simulink model "torqueBalancingStandup"  (Simulink 8.8)
settings: Solver=FixedStepDiscrete  StartTime=0.0  StopTime="Config.SIMULATION_TIME "  FixedStep=Config.Ts  RelTol=1e-3  EnableMultiTasking=on
InitFcn:
  | cd(fileparts(which(bdroot)));
  | initTorqueBalancingStandup;
StopFcn:
  | cd(fileparts(which(bdroot)));
  | stopTorqueBalancingStandup;
undefined symbols (not defined in the file or in its folder): bVectorConstraintsFeet, bVectorConstraintsLegs, Config, ConstraintsMatrixFeet, ConstraintsMatrixLegs, Gain, HUMAN_DOF_FOR_SIMULINK, Reg, ROBOT_DOF, ROBOT_DOF_FOR_SIMULINK, Sat, Sm
libraries: WBToolboxLibrary x128, simulink x4
(part 3 of 3)

== matlab function Robot System/Robot State and References/State Machine Standup/Compute base to fixed link transform/LFoot to base link transform /fromImuToHomogeousTransformFCN ==
  data: imu_H_link input double; imu_H_link_0 input double; link_H_base input double; inertial_0 input double; inertial input double; neck_pos input double; w_H_b output double; Config parameter double
function w_H_b = worldToBaseTransformWithIMUFCN(imu_H_link,imu_H_link_0,link_H_base,inertial_0,inertial,neck_pos,Config)

    w_H_b = worldToBaseTransformWithIMU(imu_H_link,imu_H_link_0,link_H_base,inertial_0,inertial,neck_pos,Config);

end

== matlab function Robot System/Dynamics and Kinematics/Kinematics/Legs in Contact ==
  data: icubStandup input double; legsInContact output double; state input double
function legsInContact = legsContactDetectorFCN(icubStandup,state)

   legsInContact = legsContactDetector(icubStandup,state);
end

== matlab function Robot System/Robot State and References/Internal Coordinator/Reference Generator CoM ==
  data: pos_CoM_0 input double; t input double; references_CoM output double; Config parameter double
function references_CoM = referenceGeneratorCoMFCN(pos_CoM_0, t, Config)

    references_CoM = referenceGeneratorCoM(pos_CoM_0, t, Config);
end

== matlab function Robot System/controller_QP/Compute angular momentum integral/Legs in Contact ==
  data: icubStandup input double; legsInContact output double; state input double
function legsInContact = legsContactDetectorFCN(icubStandup,state)

   legsInContact = legsContactDetector(icubStandup,state);
end

== matlab function Robot System/robot world to human feet transformation/MATLAB Function ==
  data: w_H_humanLeftFeet output double; w_H_robotLeftFeet input double; w_H_robotRightFeet input double; w_H_humanRightFeet output double
function [w_H_humanLeftFeet, w_H_humanRightFeet ]= fcn(w_H_robotLeftFeet,w_H_robotRightFeet)

    %% Fixed transformation from the robot feet to human feet defined
    %  human-forces-provider module configuration
    robotLeftFeet_H_humanLeftFeet = [-1.0   0.0     0.0     0.59;
                                      0.0  -1.0     0.0    -0.2549;
                                      0.0   0.0     1.0     0.0;
                                      0.0   0.0     0.0     1.0];
                                  
    robotRightFeet_H_humanRightFeet = [-1.0   0.0     0.0     0.59;
                                        0.0  -1.0     0.0    -0.2549;
                                        0.0   0.0     1.0     0.0;
                                        0.0   0.0     0.0     1.0];
                                  
    w_H_humanLeftFeet  = w_H_robotLeftFeet * robotLeftFeet_H_humanLeftFeet;
    
    w_H_humanRightFeet = w_H_robotRightFeet * robotRightFeet_H_humanRightFeet;

end

== matlab function Robot System/Robot State and References/State Machine Standup/stateMachineStandupFCN ==
  data: wrench_rightFoot input double; wrench_leftFoot input double; w_H_b output double; constraints output double; CoM_des output double; qj_des output double; wrench_leftHand input double; wrench_rightHand input double; xCoM_0 input double; qj_0 input double; xCoM input double; l_sole_H_b input double; l_upper_leg_contact_H_b input double; t input double; STANDUP_WITH_HUMAN_FORCE input double; STANDUP_WITH_HUMAN_TORQUE input double; Sm parameter double; impedances output double; KPCoM output double; KDCoM output double; Gain parameter double; currentState output double; jointsAndCoMSmoothingTime output double; fArms_phri input double
function [w_H_b, constraints, CoM_des, qj_des, impedances, KPCoM, KDCoM, currentState, jointsAndCoMSmoothingTime] = ...
             stateMachineStandupFCN(wrench_rightFoot, wrench_leftFoot, wrench_leftHand, wrench_rightHand, xCoM_0, qj_0, xCoM, l_sole_H_b, l_upper_leg_contact_H_b, t, STANDUP_WITH_HUMAN_FORCE, STANDUP_WITH_HUMAN_TORQUE, Sm, Gain, fArms_phri)
         
         [w_H_b, constraints, CoM_des, qj_des, impedances, KPCoM, KDCoM, currentState, jointsAndCoMSmoothingTime] = ...
             stateMachineStandup(wrench_rightFoot, wrench_leftFoot, wrench_leftHand, wrench_rightHand, xCoM_0, qj_0, xCoM, l_sole_H_b, l_upper_leg_contact_H_b, t, STANDUP_WITH_HUMAN_FORCE, STANDUP_WITH_HUMAN_TORQUE, Sm, Gain, fArms_phri);
end

== matlab function Robot System/Robot State and References/State Machine Standup/Compute State Velocity/Fixed Links Jacobians/Legs in Contact ==
  data: icubStandup input double; legsInContact output double; state input double
function legsInContact = legsContactDetectorFCN(icubStandup,state)

   legsInContact = legsContactDetector(icubStandup,state);
end

== matlab function Robot System/controller_QP/Balancing Controller  ==
  data: tauModel output double; Sigma output double; NA output double; f_HDot output double; HessianMatrixQP1Foot output double; gradientQP1Foot output double; ConstraintsMatrixQP1Foot output double; bVectorConstraintsQp1Foot output double; HessianMatrixQP2FeetOrLegs output double; gradientQP2FeetOrLegs output double; ConstraintsMatrixQP2FeetOrLegs output double; bVectorConstraintsQp2FeetOrLegs output double; constraints input double; ROBOT_DOF_FOR_SIMULINK input double; ConstraintsMatrix input double; bVectorConstraints input double; qj input double; qjDes input double; nu input double; M input double; h input double; H input double; intHw input double; w_H_l_contact input double; w_H_r_contact input double; JL input double; JR input double; dJL_nu input double; dJR_nu input double; xCoM input double; J_CoM input double; JComDot_nu input double; desired_x_dx_ddx_CoM input double; w_H_lArm_contact input double; w_H_rArm_contact input double; JLArm input double; JRArm input double; dJLArm_nu input double; dJRArm_nu input double; human_M input double; human_h input double; human_w_H_l_contact input double; human_w_H_r_contact input double; human_JL input double; human_JR input double; human_dJL_nu input double; human_dJR_nu input double; human_w_H_lArm_contact input double; human_w_H_rArm_contact input double; human_JLArm input double; human_JRArm input double; human_dJLArm_nu input double; human_dJRArm_nu input double; gainsPCOM input double; gainsDCOM input double; impedances input double; Reg parameter double; errorCoM output double; f_noQP output double; Gain parameter double; LArmWrench input double; RArmWrench input double; STANDUP_WITH_HUMAN_FORCE input double; STANDUP_WITH_HUMAN_TORQUE input double; correctionFromSupportForce output double; H_error output double; V output double; state input double; human_w_H_b input double; human_qj input double; human_nu_b input double; human_dqj input double; human_torques input double; HUMAN_DOF_FOR_SIMULINK input double; robot_torques input double; fArms output double; alpha output double
function [tauModel, Sigma, NA, f_HDot, ...
          HessianMatrixQP1Foot, gradientQP1Foot, ConstraintsMatrixQP1Foot, bVectorConstraintsQp1Foot, ...
          HessianMatrixQP2FeetOrLegs, gradientQP2FeetOrLegs, ConstraintsMatrixQP2FeetOrLegs, bVectorConstraintsQp2FeetOrLegs, ...
          errorCoM, f_noQP, correctionFromSupportForce, H_error, V, fArms, alpha] =  ...
              balancingControllerStandupFCN(constraints, ROBOT_DOF_FOR_SIMULINK, ConstraintsMatrix, bVectorConstraints, ...
                                            qj, qjDes, nu, M, h, H, intHw, w_H_l_contact, w_H_r_contact, JL, JR, dJL_nu, dJR_nu, xCoM, J_CoM, JComDot_nu,desired_x_dx_ddx_CoM, ...
                                            w_H_lArm_contact, w_H_rArm_contact, JLArm, JRArm, dJLArm_nu, dJRArm_nu,...
                                            human_M,human_h,...
                                            human_w_H_l_contact, human_w_H_r_contact, human_JL, human_JR, human_dJL_nu, human_dJR_nu,...
                                            human_w_H_lArm_contact, human_w_H_rArm_contact, human_JLArm, human_JRArm, human_dJLArm_nu, human_dJRArm_nu,...
                                            gainsPCOM, gainsDCOM, impedances, Reg, Gain, LArmWrench, RArmWrench, STANDUP_WITH_HUMAN_FORCE, STANDUP_WITH_HUMAN_TORQUE, state,...
                                            human_w_H_b, human_qj, human_nu_b, human_dqj, human_torques, HUMAN_DOF_FOR_SIMULINK, robot_torques)
           
   [tauModel, Sigma, NA, f_HDot, ...
          HessianMatrixQP1Foot, gradientQP1Foot, ConstraintsMatrixQP1Foot, bVectorConstraintsQp1Foot, ...
          HessianMatrixQP2FeetOrLegs, gradientQP2FeetOrLegs, ConstraintsMatrixQP2FeetOrLegs, bVectorConstraintsQp2FeetOrLegs, ...
          errorCoM, f_noQP, correctionFromSupportForce, H_error, V, fArms, alpha] =  ...
              balancingControllerStandup(constraints, ROBOT_DOF_FOR_SIMULINK, ConstraintsMatrix, bVectorConstraints, ...
                                         qj, qjDes, nu, M, h, H, intHw, w_H_l_contact, w_H_r_contact, JL, JR, dJL_nu, dJR_nu, xCoM, J_CoM, JComDot_nu, desired_x_dx_ddx_CoM, ...
                                         w_H_lArm_contact, w_H_rArm_contact, JLArm, JRArm, dJLArm_nu, dJRArm_nu,...
                                         human_M,human_h,...
                                         human_w_H_l_contact, human_w_H_r_contact, human_JL, human_JR, human_dJL_nu, human_dJR_nu,...
                                         human_w_H_lArm_contact, human_w_H_rArm_contact, human_JLArm, human_JRArm, human_dJLArm_nu, human_dJRArm_nu,...
                                         gainsPCOM, gainsDCOM, impedances, Reg, Gain, LArmWrench, RArmWrench, STANDUP_WITH_HUMAN_FORCE, STANDUP_WITH_HUMAN_TORQUE, state,...
                                         human_w_H_b, human_qj, human_nu_b, human_dqj, human_torques, HUMAN_DOF_FOR_SIMULINK, robot_torques);
end

== matlab function Robot System/emergency stop: joint limits/MATLAB Function ==
  data: umin input double; umax input double; u input double; inRange output double; tol input double
function inRange = checkRangeFCN(umin, umax, u, tol)

    inRange = checkRange(umin, umax, u, tol);
end

== matlab function Robot System/controller_QP/Compute angular momentum integral/References for H ==
  data: qjErr input double; JL input double; JR input double; nu_b_equivalent output double; Reg parameter double; activeFeetConstraints input double
function nu_b_equivalent = generateReferencesForH_FCN(qjErr, JL, JR, Reg, activeFeetConstraints)

    if activeFeetConstraints(1) == 1
    
        pinvJb          = (JL(:,1:6)'*JL(:,1:6) + Reg.pinvDamp_nu_b*eye(6))\JL(:,1:6)';
        nu_b_equivalent = -pinvJb*JL(:,7:end)*qjErr;
    else
    
        pinvJb          = (JR(:,1:6)'*JR(:,1:6) + Reg.pinvDamp_nu_b*eye(6))\JR(:,1:6)';
        nu_b_equivalent = -pinvJb*JR(:,7:end)*qjErr;
    end
end

== matlab function Robot System/Robot State and References/State Machine Standup/Visualise extrnal wrenches/Compute current threshold ==
  data: thresholdContactLeftHand output double; thresholdContactRightHand output double; state input double; thresholdContactLeftFoot output double; thresholdContactRightFoot output double; Sm parameter double
function [thresholdContactLeftHand,thresholdContactRightHand, ...
          thresholdContactLeftFoot,thresholdContactRightFoot] = currentThreshold(state,Sm)

    thresholdContactLeftHand  = Sm.wrench_thresholdContactLHand(state);
    thresholdContactRightHand = Sm.wrench_thresholdContactRHand(state);
    thresholdContactLeftFoot  = Sm.wrench_thresholdContactLFoot(state);
    thresholdContactRightFoot = Sm.wrench_thresholdContactRFoot(state);
end
